simulink model "polyinterp_3_"  (Simulink 7.8)
settings: Solver=ode45  StartTime=0.0  StopTime=2.0  RelTol=1e-3
values from neighbouring files (symbols this model uses):
  h = firpm(64,f,m)    [CFIR_1.m]    (also in adapt_filter1.m = adaptfilt.lms(ni,mu); adapt_filter2.m = adaptfilt.blms(ni,mu,1,36); adaptiv_2.m = [1 2 3 4 5 6 7 8 9 10]; adaptiv_3.m = [1 2 3 4 5 6 7 8 9 10])
  Ts = 1/fs    (= 6.25e-05)    [G722_1.m]    (also in adaptiv_2.m = 0.001; adaptiv_3.m = 0.001; adaptiv_4.m = 0.001; adaptiv_5.m = 0.001)
undefined symbols (not defined in the file or in its folder): g
libraries: dspobslib x1, dspsigops x1
settings Model: Creator=svenhoffmann  LastModifiedBy=josef  ExtModeAutoUpdateStatusClock=off
settings DataIOCC: SignalLoggingName=sigsOut
settings OptimizationCC: InitFltsAndDblsToZero=on
settings DebuggingCC: SaveWithParameterizedLinksMsg=none  SignalResolutionControl=TryResolveAllWithWarning  SolverPrmCheckMsg=none  MultiTaskDSMMsg=warning  MultiTaskCondExecSysMsg=none  FcnCallInpInsideContextMsg=Use local settings  StrictBusMsg=None
settings HardwareCC: TargetUnknown=on
settings RTWCC: IncludeERTFirstTime=on
settings GRTTargetCC: TargetFcnLib=ansi_tfl_tmw.mat

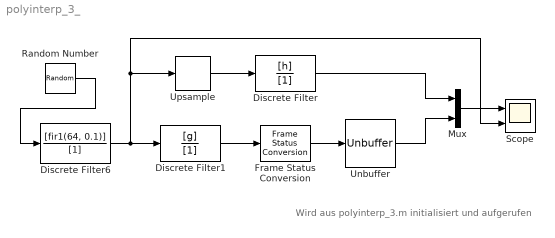
== system polyinterp_3_ ==
  note: Wird aus polyinterp_3.m initialisiert und aufgerufen
  Discrete Filter : DiscreteFilter  Numerator=[h]  Denominator=[1]  SampleTime=Ts/5
  Discrete Filter1 : DiscreteFilter  Numerator=[g]  Denominator=[1]  SampleTime=Ts
  Discrete Filter6 : DiscreteFilter  Numerator=[fir1(64, 0.1)]  Denominator=[1]  SampleTime=Ts
  Frame Status Conversion : dspobslib/Frame Status Conversion  growRefPort=off  outframe=Frame-based
  Mux : Mux  Inputs=2
  Random Number : RandomNumber  SampleTime=Ts
  Scope : Scope  NumInputPorts=2
      settings: YMin=-0.3~-15  YMax=0.35~12.5
  Unbuffer : Unbuffer
  Upsample : dspsigops/Upsample  N=5  phase=0  InputProcessing=Inherited (this choice will be removed - see release notes)  RateOptions=Allow multirate processing  ic=0  mode=Unused parameter value
  wires:
  Random Number/1 -> Discrete Filter6/1
  Discrete Filter/1 -> Mux/1
  Mux/1 -> Scope/1
  Upsample/1 -> Discrete Filter/1
  Discrete Filter6/1 -> Discrete Filter1/1, Upsample/1, Scope/2
  Unbuffer/1 -> Mux/2
  Frame Status Conversion/1 -> Unbuffer/1
  Discrete Filter1/1 -> Frame Status Conversion/1
